simulink model "ModellingStatus"  (R2021b)
settings: Solver=VariableStepAuto  StartTime=0.0  StopTime=10.0  MaxStep=0.002  RelTol=1e-3
values from neighbouring files (symbols this model uses):
  g = 9.81    [ModellingData.m]    (also in testing.m)
  l = 1    [ModellingData.m]    (also in testing.m)
  mc = 3    [ModellingData.m]    (also in testing.m)
  mp = 0.5    [ModellingData.m]    (also in testing.m)
undefined symbols (not defined in the file or in its folder): Ib, Iw, mb
settings Model: Creator=simone  LastModifiedBy=simone

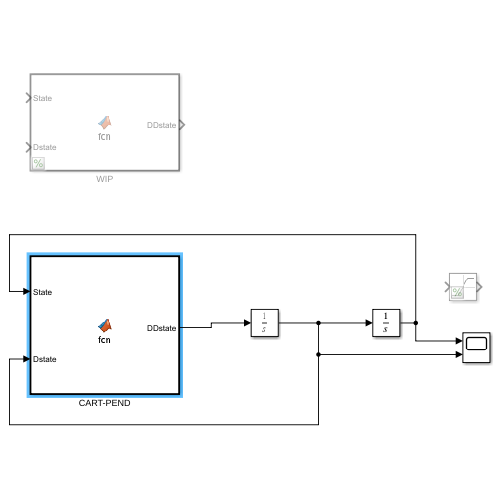
[thumbnail: Simulink's stored preview of the top-level diagram]
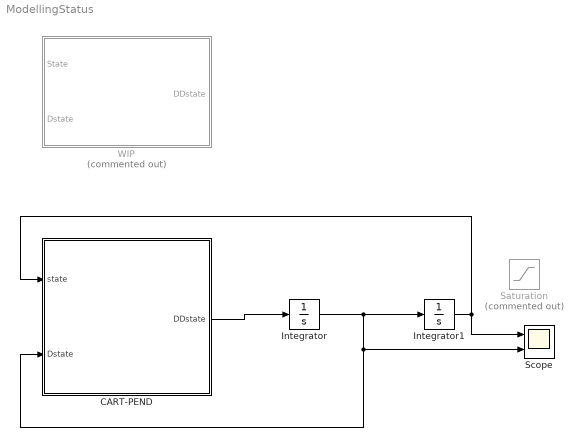
== system ModellingStatus ==
  CART-PEND : MATLAB Function  TreatAsAtomicUnit=on
  Integrator : Integrator  InitialCondition=[0;0]
  Integrator1 : Integrator  InitialCondition=[0;0.001]
  Saturation : Saturate  Commented=on  UpperLimit=[400;pi/2]  LowerLimit=[-400;-pi/2]
  Scope : Scope  NumInputPorts=2
  WIP : MATLAB Function  Commented=on  TreatAsAtomicUnit=on
  wires:
  Integrator/1 -> CART-PEND/2(Dstate), Scope/2, Integrator1/1
  Integrator1/1 -> Scope/1, CART-PEND/1(state)
  CART-PEND/1(DDstate) -> Integrator/1

== matlab function ModellingStatus/CART-PEND ==
  data: state input; DDstate output; Dstate input; g parameter; mp parameter; l parameter; mc parameter
function DDstate = fcn(state,Dstate,g, mp, l, mc)
theta=state(2);
Dtheta=Dstate(2);
F=[-31.6228,-76.4152,784.9593,401.2544]*[state;Dstate];

DDx= (- l*mp*sin(theta)*Dtheta^2 + F + g*mp*cos(theta)*sin(theta))/(- mp*cos(theta)^2 + mc + mp);
DDtheta= (- l*mp*cos(theta)*sin(theta)*Dtheta^2 + F*cos(theta) + g*mc*sin(theta) + g*mp*sin(theta))/(l*(- mp*cos(theta)^2 + mc + mp));
DDstate = [DDx;DDtheta];

end

== matlab function ModellingStatus/WIP ==
  data: State input; DDstate output; Dstate input; g parameter; Iw parameter; mb parameter; l parameter; Ib parameter
function DDstate = fcn(State,Dstate,g, Iw, mb, l, Ib)
theta=State(2);
DDpsi=1/Iw*(-mb*g*cos(theta)*l);
DDtheta=1/Ib*DDpsi;
DDstate = [DDpsi;DDtheta];
